simulink model "simple_switch_model1"  (R2023b)
settings: Solver=VariableStepAuto  StartTime=0.0  StopTime=10.0  RelTol=1e-3
settings Model: Creator=39216  LastModifiedBy=39216

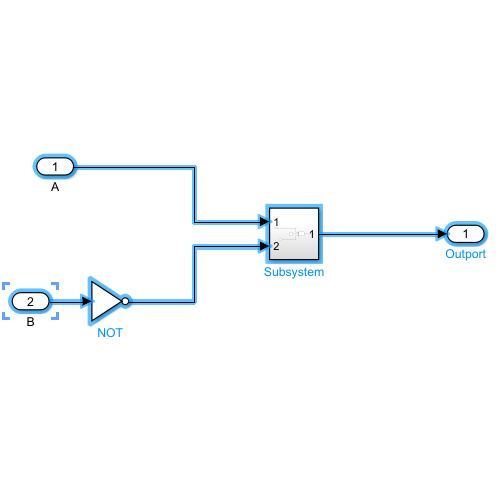
[thumbnail: Simulink's stored preview of the top-level diagram]
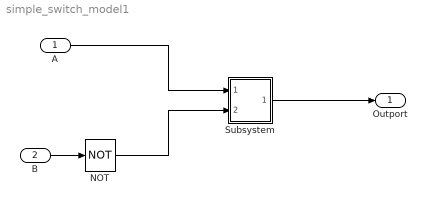
== system simple_switch_model1 ==
  A : Inport
  B : Inport  Port=2
  NOT : Logic  Operator=NOT  IconShape=distinctive  AllPortsSameDT=off  OutDataTypeStr=boolean
  Subsystem : Subsystem
  Outport : Outport
  wires:
  B/1 -> NOT/1
  A/1 -> Subsystem/1(In1)
  NOT/1 -> Subsystem/2(In2)
  Subsystem/1(Out1) -> Outport/1

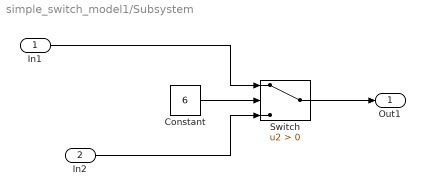
== system simple_switch_model1/Subsystem ==
  In1 : Inport
  In2 : Inport  Port=2
  Constant : Constant  Value=6
  Switch : Switch  Criteria=u2 > Threshold  SaturateOnIntegerOverflow=off  InputSameDT=off
  Out1 : Outport
  wires:
  Constant/1 -> Switch/2
  Switch/1 -> Out1/1
  In1/1 -> Switch/1
  In2/1 -> Switch/3
